simulink model "COSTEP_Auto"  (R2024b)
settings: Solver=FixedStepAuto  StartTime=0.0  StopTime=25  FixedStep=1/3600  RelTol=1e-3
model workspace (MAT data in the model file):
  AD : Simulink.Parameter (value not decoded)
  AG : Simulink.Parameter (value not decoded)
  AH : Simulink.Parameter (value not decoded)
  AV : Simulink.Parameter (value not decoded)
  AVP : Simulink.Parameter (value not decoded)
  BCHL : Simulink.Parameter (value not decoded)
  BCHV : Simulink.Parameter (value not decoded)
  BD : Simulink.Parameter (value not decoded)
  BG : Simulink.Parameter (value not decoded)
  BH : Simulink.Parameter (value not decoded)
  BVP : Simulink.Parameter (value not decoded)
  CD : Simulink.Parameter (value not decoded)
  CG : Simulink.Parameter (value not decoded)
  CH : Simulink.Parameter (value not decoded)
  CVP : Simulink.Parameter (value not decoded)
  ISV : Simulink.Parameter (value not decoded)
  XMW : Simulink.Parameter (value not decoded)
  XNS : Simulink.Parameter (value not decoded)
  XNS2 : Simulink.Parameter (value not decoded)
  XNS3 : Simulink.Parameter (value not decoded)
  XNSE : Simulink.Parameter (value not decoded)
values from neighbouring files (symbols this model uses):
  DD = SimData{4,1}{1,2}    [Auto_run_COSTEP.m]    (also in Run_COSTEP.m)
  G = SimData{2,1}(j,2)    [Auto_run_COSTEP.m]    (also in G.mat = [4243534565 7854912354 3456432354 1731738903 4346024432 5784; Run_COSTEP.m)
  IDV = SimData{3,1}(1:20,j)    [Auto_run_COSTEP.m]    (also in IDV.mat = [0 0 0 0 0 0 0 0 0 0 0 0 ... (812 elements, 28x29)]; Run_COSTEP.m = SimData{3,1}(1:28,j))
symbols that are objects in the model workspace (value not decoded): AD, AG, AH, AV, AVP, BD, BG, BH, BVP, CD, CG, CH, CVP, XMW, XNS, XNS2, XNS3, XNSE
undefined symbols (not defined in the file or in its folder): magnitude, msgbox, SETPT, XMEAS, XMV
libraries: mylib x304, dspindex x31
(part 7 of 13)

== system COSTEP_Auto/Stream Measurements/Subsystem6/E feed stream ==
  Stream 2 : Inport
  Bus Creator : BusCreator  Inputs=4
  Bus Selector : BusSelector  OutputSignals=XMNSE(3),XMNSE(4)
  Bus Selector1 : BusSelector  OutputSignals=TST(2),XST(I;2)
  Bus Selector2 : BusSelector  OutputSignals=Stream 2
  Bus Selector3 : BusSelector  OutputSignals=signal1.XMEAS(3)
  Composition measurement mol% : Subsystem
  Constant : Constant  Value=1000
  Flow measurement in kg/h : Subsystem
  Pressure measurement in kPa : Subsystem
  Temperature measurement in C : Subsystem
  tag scope: SM3=global
  wires:
  Bus Selector1/1 -> Temperature measurement in C/1(T in celsius)  "<TST(2)>"
  Temperature measurement in C/1(SMEAST(3)) -> Bus Creator/1  "SMEAST(3)"
  [XMNSE] -> Bus Selector/1
  Bus Selector/1 -> Temperature measurement in C/2(XMNSE)  "<XMNSE(3)>"
  Bus Selector/2 -> Pressure measurement in kPa/2(XMNSE)  "<XMNSE(4)>"
  Stream 2/1 -> Bus Selector1/1
  Bus Selector1/2 -> Composition measurement mol%/1(XST)  "<XST(I;2)>"
  Constant/1 -> Pressure measurement in kPa/1("P in mm Hg ")
  Pressure measurement in kPa/1(SMEASP(3)) -> Bus Creator/2  "SMEASP(3)"
  Flow measurement in kg/h/1("SMEASF(3) ") -> Bus Creator/3  "SMEASF(3)"
  Composition measurement mol%/1(SMEASX(3)) -> Bus Creator/4  "SMEASX(3)"
  Bus Creator/1 -> [SM3]
  [XMNSE2] -> Bus Selector2/1
  Bus Selector2/1 -> Composition measurement mol%/2(XMNSE)  "<Stream 2>"
  [XMEAS] -> Bus Selector3/1
  Bus Selector3/1 -> Flow measurement in kg/h/1(XMEAS in kg/h)  "<XMEAS(3)>"

== system COSTEP_Auto/Stream Measurements/Subsystem6/Product stream ==
  Stream 13 : Inport
  Bus Creator : BusCreator  Inputs=4
  Bus Selector : BusSelector  OutputSignals=XMNSE(14)
  Bus Selector1 : BusSelector  OutputSignals=PTC,XST(I;13)
  Bus Selector2 : BusSelector  OutputSignals=Stream 13
  Bus Selector3 : BusSelector  OutputSignals=signal4.XMEAS(18),signal4.XMEAS(17)
  Bus Selector4 : BusSelector  OutputSignals=Stream 13
  Composition measurement mol% : Subsystem
  Flow measurement in kg/h : Subsystem
  Pressure measurement in kPa : Subsystem
  Temperature measurement in C : Subsystem
  tag scope: SM11=global
  wires:
  Temperature measurement in C/1(SMEAST) -> Bus Creator/1
  [XMNSE] -> Bus Selector/1
  Stream 13/1 -> Bus Selector1/1
  Pressure measurement in kPa/1(SMEASP) -> Bus Creator/2
  Flow measurement in kg/h/1("SMEASF ") -> Bus Creator/3  "SMEASF"
  Composition measurement mol%/1(SMEASX) -> Bus Creator/4
  Bus Creator/1 -> [SM11]
  [XMNSE2] -> Bus Selector2/1
  Bus Selector2/1 -> Composition measurement mol%/2(XMNSE2)  "<Stream 13>"
  [XMEAS] -> Bus Selector3/1
  Bus Selector/1 -> Pressure measurement in kPa/2(XMNSE)  "<XMNSE(14)>"
  Bus Selector1/1 -> Pressure measurement in kPa/1("P in mm Hg ")  "<PTC>"
  Bus Selector3/1 -> Temperature measurement in C/1(XMEAS in celsius)  "<XMEAS(18)>"
  Bus Selector3/2 -> Flow measurement in kg/h/1(XMEAS in m^3/h)  "<XMEAS(17)>"
  Bus Selector1/2 -> Composition measurement mol%/1(XST), Flow measurement in kg/h/2(XST)  "<XST(I;13)>"
  [XMNSE3] -> Bus Selector4/1
  Bus Selector4/1 -> Composition measurement mol%/3(XMNSE3)  "<Stream 13>"

== system COSTEP_Auto/Stream Measurements/Subsystem6/Purge stream ==
  Stream 10 : Inport
  Bus Creator : BusCreator  Inputs=4
  Bus Selector : BusSelector  OutputSignals=XMNSE(2)
  Bus Selector1 : BusSelector  OutputSignals=signal1.XST(I;10)
  Bus Selector3 : BusSelector  OutputSignals=signal3.XMEAS(11),signal3.XMEAS(10),signal9
  Composition measurement mol% : Subsystem
  Flow measurement in kg/h : Subsystem
  Pressure measurement in kPa : Subsystem
  Temperature measurement in C : Subsystem
  tag scope: SM9=global
  wires:
  Temperature measurement in C/1(SMEAST) -> Bus Creator/1  "SMEAST"
  Stream 10/1 -> Bus Selector1/1
  Bus Selector1/1 -> Flow measurement in kg/h/2(XST)  "<XST(I;10)>"
  Pressure measurement in kPa/1(SMEASP) -> Bus Creator/2
  Flow measurement in kg/h/1("SMEASF ") -> Bus Creator/3  "SMEASF"
  Composition measurement mol%/1(SMEASX) -> Bus Creator/4
  Bus Creator/1 -> [SM9]
  [XMEAS] -> Bus Selector3/1
  Bus Selector3/1 -> Temperature measurement in C/1(XMEAS in celsius)  "<XMEAS(11)>"
  Bus Selector3/2 -> Flow measurement in kg/h/1(XMEAS in kscmh)  "<XMEAS(10)>"
  Bus Selector3/3 -> Composition measurement mol%/1(XMEAS)  "<signal9>"
  [XMNSE] -> Bus Selector/1
  Bus Selector/1 -> Pressure measurement in kPa/1(XMNSE)  "<XMNSE(2)>"

== system COSTEP_Auto/Stream Measurements/Subsystem6/RCIn ==
  Bus Creator : BusCreator  Inputs=3
  Bus Selector : BusSelector  OutputSignals=XMNSE(15),XMNSE(16),XMNSE(17)
  Flow measurement in kg/h : Subsystem
  Pressure measurement in kPa : Subsystem
  Temperature measurement in C : Subsystem
  tag scope: SM16=global
  wires:
  [TCWR] -> Pressure measurement in kPa/2(TC), Temperature measurement in C/1(T in celsius)
  [FWR] -> Flow measurement in kg/h/2(F in gpm)
  [XMNSE] -> Bus Selector/1
  Bus Selector/1 -> Temperature measurement in C/2(XMNSE)  "<XMNSE(15)>"
  Bus Selector/2 -> Pressure measurement in kPa/1(XMNSE)  "<XMNSE(16)>"
  Bus Selector/3 -> Flow measurement in kg/h/1(XMNSE)  "<XMNSE(17)>"
  Temperature measurement in C/1(SMEAST) -> Bus Creator/1
  Pressure measurement in kPa/1(SMEASP) -> Bus Creator/2
  Flow measurement in kg/h/1("SMEASF ") -> Bus Creator/3
  Bus Creator/1 -> [SM16]

== system COSTEP_Auto/Stream Measurements/Subsystem6/RCOut ==
  Bus Creator : BusCreator  Inputs=2
  Bus Selector : BusSelector  OutputSignals=XMNSE(18),XMNSE(19)
  Pressure measurement in kPa : Subsystem
  Temperature measurement in C : Subsystem
  tag scope: SM12=global
  wires:
  [TWR] -> Pressure measurement in kPa/2(TC), Temperature measurement in C/1(T in celsius)
  Bus Creator/1 -> [SM12]
  [XMNSE] -> Bus Selector/1
  Bus Selector/1 -> Temperature measurement in C/2(XMNSE)  "<XMNSE(18)>"
  Bus Selector/2 -> Pressure measurement in kPa/1(XMNSE)  "<XMNSE(19)>"
  Temperature measurement in C/1(SMEAST) -> Bus Creator/1
  Pressure measurement in kPa/1(SMEASP) -> Bus Creator/2

== system COSTEP_Auto/Stream Measurements/Subsystem6/Reactor feed stream ==
  Stream 6 : Inport
  Bus Creator : BusCreator  Inputs=4
  Bus Selector : BusSelector  OutputSignals=XMNSE(11)
  Bus Selector1 : BusSelector  OutputSignals=signal1.TST(6) = TST(7),signal1.XST(I;6) = XST(I;7)
  Bus Selector2 : BusSelector  OutputSignals=Stream 6
  Bus Selector3 : BusSelector  OutputSignals=signal4.XMEAS(16),signal2.XMEAS(6),signal8
  Composition measurement mol% : Subsystem
  Flow measurement in kg/h : Subsystem
  Pressure measurement in kPa : Subsystem
  Temperature measurement in C : Subsystem
  tag scope: SM6=global
  wires:
  Bus Selector1/1 -> Temperature measurement in C/1(T in celsius)  "<TST(6) = TST(7)>"
  Temperature measurement in C/1(SMEAST) -> Bus Creator/1  "SMEAST(6)"
  [XMNSE] -> Bus Selector/1
  Bus Selector/1 -> Temperature measurement in C/2(XMNSE)  "<XMNSE(11)>"
  Stream 6/1 -> Bus Selector1/1
  Bus Selector1/2 -> Flow measurement in kg/h/2(XST), Composition measurement mol%/1(XST)  "<XST(I;6) = XST(I;7)>"
  [XMEAS] -> Bus Selector3/1
  Pressure measurement in kPa/1(SMEASP) -> Bus Creator/2  "SMEASP(6)"
  Flow measurement in kg/h/1("SMEASF ") -> Bus Creator/3  "SMEASF(6)"
  Composition measurement mol%/1(SMEASX(6)) -> Bus Creator/4  "SMEASX(6)"
  Bus Creator/1 -> [SM6]
  [XMNSE2] -> Bus Selector2/1
  Bus Selector2/1 -> Composition measurement mol%/2(XMNSE)  "<Stream 6>"
  Bus Selector3/1 -> Pressure measurement in kPa/1(XMEAS in kPa gauge)  "<XMEAS(16)>"
  Bus Selector3/2 -> Flow measurement in kg/h/1(XMEAS in kscmh)  "<XMEAS(6)>"
  Bus Selector3/3 -> Composition measurement mol%/3(XMEAS)  "<signal8>"

== system COSTEP_Auto/Stream Measurements/Subsystem6/Reactor product stream ==
  Stream 8 : Inport
  Bus Creator : BusCreator  Inputs=4
  Bus Selector : BusSelector  OutputSignals=XMNSE(12)
  Bus Selector1 : BusSelector  OutputSignals=signal1.XST(I;8),signal1.FTM(8)
  Bus Selector2 : BusSelector  OutputSignals=Stream 8
  Bus Selector3 : BusSelector  OutputSignals=signal2.XMEAS(9),signal2.XMEAS(7)
  Composition measurement mol% : Subsystem
  Flow measurement in kg/h : Subsystem
  Pressure measurement in kPa : Subsystem
  Temperature measurement in C : Subsystem
  tag scope: SM7=global
  wires:
  Temperature measurement in C/1(SMEAST) -> Bus Creator/1
  [XMNSE] -> Bus Selector/1
  Stream 8/1 -> Bus Selector1/1
  Bus Selector1/1 -> Composition measurement mol%/1(XST), Flow measurement in kg/h/1(XST)  "<XST(I;8)>"
  Pressure measurement in kPa/1(SMEASP) -> Bus Creator/2
  Flow measurement in kg/h/1("SMEASF ") -> Bus Creator/3
  Composition measurement mol%/1(SMEASX) -> Bus Creator/4
  Bus Creator/1 -> [SM7]
  [XMNSE2] -> Bus Selector2/1
  Bus Selector2/1 -> Composition measurement mol%/2(XMNSE)  "<Stream 8>"
  [XMEAS] -> Bus Selector3/1
  Bus Selector3/1 -> Temperature measurement in C/1(XMEAS in celsius)  "<XMEAS(9)>"
  Bus Selector3/2 -> Pressure measurement in kPa/1(XMEAS in kPa gauge)  "<XMEAS(7)>"
  Bus Selector1/2 -> Flow measurement in kg/h/3(F in lb-mol/h)  "<FTM(8)>"
  Bus Selector/1 -> Flow measurement in kg/h/2(XMNSE)  "<XMNSE(12)>"

== system COSTEP_Auto/Stream Measurements/Subsystem6/Separator product stream ==
  Stream 9 : Inport
  Bus Creator : BusCreator  Inputs=4
  Bus Selector1 : BusSelector  OutputSignals=signal2.XST(I;9)
  Bus Selector2 : BusSelector  OutputSignals=Stream 9
  Bus Selector3 : BusSelector  OutputSignals=signal3.XMEAS(11),signal3.XMEAS(13),signal1.XMEAS(5),signal3.XMEAS(10)
  Composition measurement mol% : Subsystem
  Flow measurement in kg/h : Subsystem
  Pressure measurement in kPa : Subsystem
  Temperature measurement in C : Subsystem
  tag scope: SMNA=global
  wires:
  Temperature measurement in C/1(SMEAST) -> Bus Creator/1  "SMEAST"
  Stream 9/1 -> Bus Selector1/1
  Bus Selector1/1 -> Flow measurement in kg/h/2(XST), Composition measurement mol%/1(XST)  "<XST(I;9)>"
  Pressure measurement in kPa/1(SMEASP) -> Bus Creator/2
  Flow measurement in kg/h/1("SMEASF ") -> Bus Creator/3  "SMEASF"
  Composition measurement mol%/1(SMEASX) -> Bus Creator/4
  Bus Creator/1 -> [SMNA]
  [XMNSE2] -> Bus Selector2/1
  Bus Selector2/1 -> Composition measurement mol%/2(XMNSE)  "<Stream 9>"
  [XMEAS] -> Bus Selector3/1
  Bus Selector3/1 -> Temperature measurement in C/1(XMEAS in celsius)  "<XMEAS(11)>"
  Bus Selector3/2 -> Pressure measurement in kPa/1(XMEAS in kPa gauge)  "<XMEAS(13)>"
  Bus Selector3/3 -> Flow measurement in kg/h/1(XMEAS in kscmh)  "<XMEAS(5)>"
  Bus Selector3/4 -> Flow measurement in kg/h/3(XMEAS in kscmh1)  "<XMEAS(10)>"

== system COSTEP_Auto/Stream Measurements/Subsystem6/Separator recycle stream (after compressor) ==
  Stream 9 : Inport
  Bus Creator : BusCreator  Inputs=4
  Bus Selector1 : BusSelector  OutputSignals=signal2.XST(I;9),signal2.HST(9),signal2.Phase
  Bus Selector2 : BusSelector  OutputSignals=Stream 9
  Bus Selector3 : BusSelector  OutputSignals=signal4.XMEAS(16),signal1.XMEAS(5)
  Composition measurement mol% : Subsystem
  Flow measurement in kg/h : Subsystem
  Pressure measurement in kPa : Subsystem
  Temperature measurement in C : Subsystem
  tag scope: SM8=global
  wires:
  Temperature measurement in C/1(SMEAST) -> Bus Creator/1  "SMEAST"
  Stream 9/1 -> Bus Selector1/1
  Bus Selector1/1 -> Temperature measurement in C/2(XST), Flow measurement in kg/h/2(XST), Composition measurement mol%/1(XST)  "<XST(I;9)>"
  Pressure measurement in kPa/1(SMEASP) -> Bus Creator/2
  Flow measurement in kg/h/1("SMEASF ") -> Bus Creator/3  "SMEASF"
  Composition measurement mol%/1(SMEASX) -> Bus Creator/4
  Bus Creator/1 -> [SM8]
  [XMNSE2] -> Bus Selector2/1
  Bus Selector2/1 -> Composition measurement mol%/2(XMNSE)  "<Stream 9>"
  [XMEAS] -> Bus Selector3/1
  Bus Selector3/1 -> Pressure measurement in kPa/1(XMEAS in kPa gauge)  "<XMEAS(16)>"
  Bus Selector3/2 -> Flow measurement in kg/h/1(XMEAS in kscmh)  "<XMEAS(5)>"
  Bus Selector1/2 -> Temperature measurement in C/1(HST(9))  "<HST(9)>"
  Bus Selector1/3 -> Temperature measurement in C/3(ITY)  "<Phase>"

== system COSTEP_Auto/Stream Measurements/Subsystem6/Separator recycle stream (before compressor) ==
  Stream 9 : Inport
  Bus Creator : BusCreator  Inputs=4
  Bus Selector1 : BusSelector  OutputSignals=signal2.XST(I;9)
  Bus Selector2 : BusSelector  OutputSignals=Stream 9
  Bus Selector3 : BusSelector  OutputSignals=signal3.XMEAS(11),signal3.XMEAS(13),signal1.XMEAS(5)
  Composition measurement mol% : Subsystem
  Flow measurement in kg/h : Subsystem
  Pressure measurement in kPa : Subsystem
  Temperature measurement in C : Subsystem
  tag scope: SM15=global
  wires:
  Temperature measurement in C/1(SMEAST) -> Bus Creator/1  "SMEAST"
  Stream 9/1 -> Bus Selector1/1
  Bus Selector1/1 -> Flow measurement in kg/h/2(XST), Composition measurement mol%/1(XST)  "<XST(I;9)>"
  Pressure measurement in kPa/1(SMEASP) -> Bus Creator/2
  Flow measurement in kg/h/1("SMEASF ") -> Bus Creator/3  "SMEASF"
  Composition measurement mol%/1(SMEASX) -> Bus Creator/4
  Bus Creator/1 -> [SM15]
  [XMNSE2] -> Bus Selector2/1
  Bus Selector2/1 -> Composition measurement mol%/2(XMNSE)  "<Stream 9>"
  [XMEAS] -> Bus Selector3/1
  Bus Selector3/1 -> Temperature measurement in C/1(XMEAS in celsius)  "<XMEAS(11)>"
  Bus Selector3/2 -> Pressure measurement in kPa/1(XMEAS in kPa gauge)  "<XMEAS(13)>"
  Bus Selector3/3 -> Flow measurement in kg/h/1(XMEAS in kscmh)  "<XMEAS(5)>"

== system COSTEP_Auto/Stream Measurements/Subsystem6/Separator underflow stream ==
  Stream 11 : Inport
  Bus Creator : BusCreator  Inputs=4
  Bus Selector1 : BusSelector  OutputSignals=signal1.PTSL,signal1.XST(I;11)
  Bus Selector2 : BusSelector  OutputSignals=Stream 11
  Bus Selector3 : BusSelector  OutputSignals=signal3.XMEAS(11),signal3.XMEAS(14)
  Bus Selector4 : BusSelector  OutputSignals=XMNSE(13)
  Composition measurement mol% : Subsystem
  Flow measurement in kg/h : Subsystem
  Pressure measurement in kPa : Subsystem
  Temperature measurement in C : Subsystem
  tag scope: SM10=global
  wires:
  Temperature measurement in C/1(SMEAST) -> Bus Creator/1
  [XMNSE] -> Bus Selector4/1
  Stream 11/1 -> Bus Selector1/1
  Pressure measurement in kPa/1(SMEASP) -> Bus Creator/2
  Flow measurement in kg/h/1("SMEASF ") -> Bus Creator/3  "SMEASF"
  Composition measurement mol%/1(SMEASX) -> Bus Creator/4
  Bus Creator/1 -> [SM10]
  [XMNSE3] -> Bus Selector2/1
  Bus Selector2/1 -> Composition measurement mol%/2(XMNSE)  "<Stream 11>"
  [XMEAS] -> Bus Selector3/1
  Bus Selector4/1 -> Pressure measurement in kPa/2(XMNSE)  "<XMNSE(13)>"
  Bus Selector1/1 -> Pressure measurement in kPa/1("P in mm Hg ")  "<PTSL>"
  Bus Selector1/2 -> Flow measurement in kg/h/2(XST), Composition measurement mol%/1(XST)  "<XST(I;11)>"
  Bus Selector3/1 -> Temperature measurement in C/1(XMEAS in celsius)  "<XMEAS(11)>"
  Bus Selector3/2 -> Flow measurement in kg/h/1(XMEAS in m^3/h)  "<XMEAS(14)>"

== system COSTEP_Auto/Stream Measurements/Subsystem6/Stripper recycle stream ==
  Stream 5 : Inport
  Bus Creator : BusCreator  Inputs=4
  Bus Selector : BusSelector  OutputSignals=XMNSE(9),XMNSE(10)
  Bus Selector1 : BusSelector  OutputSignals=TST(5),XST(I;5),FTM(5)
  Bus Selector2 : BusSelector  OutputSignals=Stream 5
  Bus Selector3 : BusSelector  OutputSignals=signal4.XMEAS(16)
  Composition measurement mol% : Subsystem
  Flow measurement in kg/h : Subsystem
  Pressure measurement in kPa : Subsystem
  Temperature measurement in C : Subsystem
  tag scope: SM5=global
  wires:
  Bus Selector1/1 -> Temperature measurement in C/1(T in celsius)  "<TST(5)>"
  Temperature measurement in C/1(SMEAST(5)) -> Bus Creator/1  "SMEAST(5)"
  [XMNSE] -> Bus Selector/1
  Bus Selector/1 -> Temperature measurement in C/2(XMNSE)  "<XMNSE(9)>"
  Stream 5/1 -> Bus Selector1/1
  Bus Selector1/2 -> Composition measurement mol%/1(XST), Flow measurement in kg/h/1(XST)  "<XST(I;5)>"
  [XMEAS] -> Bus Selector3/1
  Pressure measurement in kPa/1(SMEASP(5)) -> Bus Creator/2  "SMEASP(5)"
  Flow measurement in kg/h/1("SMEASF(5) ") -> Bus Creator/3  "SMEASF(5)"
  Composition measurement mol%/1(SMEASX(5)) -> Bus Creator/4  "SMEASX(5)"
  Bus Creator/1 -> [SM5]
  [XMNSE2] -> Bus Selector2/1
  Bus Selector2/1 -> Composition measurement mol%/2(XMNSE)  "<Stream 5>"
  Bus Selector3/1 -> Pressure measurement in kPa/1(XMEAS in kPa gauge)  "<XMEAS(16)>"
  Bus Selector1/3 -> Flow measurement in kg/h/3(F in lb-mol/h)  "<FTM(5)>"
  Bus Selector/2 -> Flow measurement in kg/h/2(XMNSE)  "<XMNSE(10)>"

== system COSTEP_Auto/Stripper/Heat transfer of stripper/If Action Subsystem ==
  In1 : Inport
  Action Port : ActionPort  ActionPortLabel=if(u1 < 100)
  Out1 : Outport  VectorParamsAs1DForOutWhenUnconnected=off
  wires:
  In1/1 -> Out1/1

== system COSTEP_Auto/Stripper/Heat transfer of stripper/If Action Subsystem1 ==
  In1 : Inport
  Action Port : ActionPort  ActionPortLabel=else
  Out1 : Outport  VectorParamsAs1DForOutWhenUnconnected=off
  wires:
  In1/1 -> Out1/1

== system COSTEP_Auto/Stripper/Holdup of Components in Stripper/Holsup of Liquid Components in Stripper ==
  YY(19:26) : Inport
  Bus Creator : BusCreator  Inputs=8
  Bus Selector : BusSelector  OutputSignals=YY(19),YY(20),YY(21),YY(22),YY(23),YY(24),YY(25),YY(26)
  UCLC(1) Holdup of Component A (Liquid) in Stripper lb-mol : Gain
  UCLC(2) Holdup of Component B (Liquid) in Stripper lb-mol : Gain
  UCLC(3) Holdup of Component C (Liquid) in Stripper lb-mol : Gain
  UCLC(4) Holdup of Component D (Liquid) in Stripper lb-mol : Gain
  UCLC(5) Holdup of Component E (Liquid) in Stripper lb-mol : Gain
  UCLC(6) Holdup of Component F (Liquid) in Stripper lb-mol : Gain
  UCLC(7) Holdup of Component G (Liquid) in Stripper lb-mol : Gain
  UCLC(8) Holdup of Component H (Liquid) in Stripper lb-mol : Gain
  UCLC : Outport  VectorParamsAs1DForOutWhenUnconnected=off
  wires:
  UCLC(8) Holdup of Component H (Liquid) in Stripper lb-mol/1 -> Bus Creator/8
  UCLC(2) Holdup of Component B (Liquid) in Stripper lb-mol/1 -> Bus Creator/2
  UCLC(1) Holdup of Component A (Liquid) in Stripper lb-mol/1 -> Bus Creator/1
  Bus Creator/1 -> UCLC/1
  UCLC(5) Holdup of Component E (Liquid) in Stripper lb-mol/1 -> Bus Creator/5
  UCLC(7) Holdup of Component G (Liquid) in Stripper lb-mol/1 -> Bus Creator/7
  UCLC(4) Holdup of Component D (Liquid) in Stripper lb-mol/1 -> Bus Creator/4
  UCLC(6) Holdup of Component F (Liquid) in Stripper lb-mol/1 -> Bus Creator/6
  UCLC(3) Holdup of Component C (Liquid) in Stripper lb-mol/1 -> Bus Creator/3
  YY(19:26)/1 -> Bus Selector/1
  Bus Selector/1 -> UCLC(1) Holdup of Component A (Liquid) in Stripper lb-mol/1  "<YY(19)>"
  Bus Selector/2 -> UCLC(2) Holdup of Component B (Liquid) in Stripper lb-mol/1  "<YY(20)>"
  Bus Selector/3 -> UCLC(3) Holdup of Component C (Liquid) in Stripper lb-mol/1  "<YY(21)>"
  Bus Selector/4 -> UCLC(4) Holdup of Component D (Liquid) in Stripper lb-mol/1  "<YY(22)>"
  Bus Selector/5 -> UCLC(5) Holdup of Component E (Liquid) in Stripper lb-mol/1  "<YY(23)>"
  Bus Selector/6 -> UCLC(6) Holdup of Component F (Liquid) in Stripper lb-mol/1  "<YY(24)>"
  Bus Selector/7 -> UCLC(7) Holdup of Component G (Liquid) in Stripper lb-mol/1  "<YY(25)>"
  Bus Selector/8 -> UCLC(8) Holdup of Component H (Liquid) in Stripper lb-mol/1  "<YY(26)>"

== system COSTEP_Auto/Stripper/Holdup of Components in Stripper/Liquid Component Fraction in Stripper ==
  UTLC : Inport
  UCLC : Inport  Port=2
  Bus Selector : BusSelector  OutputSignals=signal1,signal2,signal3,signal4,signal5,signal6,signal7,signal8
  Mux : Mux  Inputs=8
  XLC(1) : Product  Inputs=*/
  XLC(2) : Product  Inputs=*/
  XLC(3) : Product  Inputs=*/
  XLC(4) : Product  Inputs=*/
  XLC(5) : Product  Inputs=*/
  XLC(6) : Product  Inputs=*/
  XLC(7) : Product  Inputs=*/
  XLC(8) : Product  Inputs=*/
  XLC : Outport  VectorParamsAs1DForOutWhenUnconnected=off
  wires:
  XLC(3)/1 -> Mux/3  "XLC(3)"
  Bus Selector/2 -> XLC(2)/1  "<signal2>"
  Bus Selector/7 -> XLC(7)/1  "<signal7>"
  XLC(5)/1 -> Mux/5  "XLC(5)"
  XLC(7)/1 -> Mux/7  "XLC(7)"
  Bus Selector/3 -> XLC(3)/1  "<signal3>"
  UTLC/1 -> XLC(8)/2, XLC(7)/2, XLC(6)/2, XLC(5)/2, XLC(4)/2, XLC(3)/2, XLC(2)/2, XLC(1)/2
  Bus Selector/6 -> XLC(6)/1  "<signal6>"
  Bus Selector/5 -> XLC(5)/1  "<signal5>"
  XLC(2)/1 -> Mux/2  "XLC(2)"
  XLC(6)/1 -> Mux/6  "XLC(6)"
  Bus Selector/4 -> XLC(4)/1  "<signal4>"
  XLC(1)/1 -> Mux/1  "XLC(1)"
  XLC(8)/1 -> Mux/8  "XLC(8)"
  UCLC/1 -> Bus Selector/1
  XLC(4)/1 -> Mux/4  "XLC(4)"
  Mux/1 -> XLC/1
  Bus Selector/1 -> XLC(1)/1  "<signal1>"
  Bus Selector/8 -> XLC(8)/1  "<signal8>"

== system COSTEP_Auto/Stripper/Holdup of Components in Stripper/YP(19) ==
  FCM(1,12) : Inport
  FCM(1,13) : Inport  Port=2
  " " : Sum  Inputs=+-
  Integration : mylib/Integration  SystemSampleTime=-1  VariantActivationTime=update diagram  AllowFlexibleInterface=on  Latency=0  AutoFrameSizeCalculation=off
  "YY(19) " : Constant  Value=0.4306056376
  YY(19) : Outport  VectorParamsAs1DForOutWhenUnconnected=off
  wires:
  "YY(19) "/1 -> Integration/2
  FCM(1,13)/1 -> " "/2
  FCM(1,12)/1 -> " "/1
  " "/1 -> Integration/1
  Integration/1 -> YY(19)/1

== system COSTEP_Auto/Stripper/Holdup of Components in Stripper/YP(20) ==
  FCM(2,12) : Inport
  FCM(2,13) : Inport  Port=2
  " " : Sum  Inputs=+-
  Integration : mylib/Integration  SystemSampleTime=-1  VariantActivationTime=update diagram  AllowFlexibleInterface=on  Latency=0  AutoFrameSizeCalculation=off
  "YY(20) " : Constant  Value=7.9906200783E-3
  YY(20) : Outport  VectorParamsAs1DForOutWhenUnconnected=off
  wires:
  Integration/1 -> YY(20)/1
  FCM(2,12)/1 -> " "/1
  FCM(2,13)/1 -> " "/2
  "YY(20) "/1 -> Integration/2
  " "/1 -> Integration/1

== system COSTEP_Auto/Stripper/Holdup of Components in Stripper/YP(21) ==
  FCM(3,12) : Inport
  FCM(3,13) : Inport  Port=2
  " " : Sum  Inputs=+-
  Integration : mylib/Integration  SystemSampleTime=-1  VariantActivationTime=update diagram  AllowFlexibleInterface=on  Latency=0  AutoFrameSizeCalculation=off
  "YY(21) " : Constant  Value=0.9056036089
  YY(21) : Outport  VectorParamsAs1DForOutWhenUnconnected=off
  wires:
  Integration/1 -> YY(21)/1
  FCM(3,12)/1 -> " "/1
  FCM(3,13)/1 -> " "/2
  " "/1 -> Integration/1
  "YY(21) "/1 -> Integration/2

== system COSTEP_Auto/Stripper/Holdup of Components in Stripper/YP(22) ==
  FCM(4,12) : Inport
  FCM(4,13) : Inport  Port=2
  " " : Sum  Inputs=+-
  Integration : mylib/Integration  SystemSampleTime=-1  VariantActivationTime=update diagram  AllowFlexibleInterface=on  Latency=0  AutoFrameSizeCalculation=off
  "YY(22) " : Constant  Value=1.6054258216E-2
  "YY(22)  " : Outport  VectorParamsAs1DForOutWhenUnconnected=off
  wires:
  Integration/1 -> "YY(22)  "/1
  FCM(4,12)/1 -> " "/1
  FCM(4,13)/1 -> " "/2
  " "/1 -> Integration/1
  "YY(22) "/1 -> Integration/2

== system COSTEP_Auto/Stripper/Holdup of Components in Stripper/YP(23) ==
  FCM(5,12) : Inport
  FCM(5,13) : Inport  Port=2
  " " : Sum  Inputs=+-
  Integration : mylib/Integration  SystemSampleTime=-1  VariantActivationTime=update diagram  AllowFlexibleInterface=on  Latency=0  AutoFrameSizeCalculation=off
  "YY(23) " : Constant  Value=0.7509759687
  "YY(23)  " : Outport  VectorParamsAs1DForOutWhenUnconnected=off
  wires:
  Integration/1 -> "YY(23)  "/1
  FCM(5,12)/1 -> " "/1
  FCM(5,13)/1 -> " "/2
  " "/1 -> Integration/1
  "YY(23) "/1 -> Integration/2

== system COSTEP_Auto/Stripper/Holdup of Components in Stripper/YP(24) ==
  FCM(6,12) : Inport
  FCM(6,13) : Inport  Port=2
  " " : Sum  Inputs=+-
  Integration : mylib/Integration  SystemSampleTime=-1  VariantActivationTime=update diagram  AllowFlexibleInterface=on  Latency=0  AutoFrameSizeCalculation=off
  YY(24) : Constant  Value=8.8582855955E-2
  "YY(24)  " : Outport  VectorParamsAs1DForOutWhenUnconnected=off
  wires:
  Integration/1 -> "YY(24)  "/1
  FCM(6,12)/1 -> " "/1
  FCM(6,13)/1 -> " "/2
  " "/1 -> Integration/1
  YY(24)/1 -> Integration/2

== system COSTEP_Auto/Stripper/Holdup of Components in Stripper/YP(25) ==
  FCM(7,12) : Inport
  FCM(7,13) : Inport  Port=2
  " " : Sum  Inputs=+-
  Integration : mylib/Integration  SystemSampleTime=-1  VariantActivationTime=update diagram  AllowFlexibleInterface=on  Latency=0  AutoFrameSizeCalculation=off
  "YY(25) " : Constant  Value=48.27726193
  "YY(25)  " : Outport  VectorParamsAs1DForOutWhenUnconnected=off
  wires:
  Integration/1 -> "YY(25)  "/1
  FCM(7,12)/1 -> " "/1
  FCM(7,13)/1 -> " "/2
  " "/1 -> Integration/1
  "YY(25) "/1 -> Integration/2

== system COSTEP_Auto/Stripper/Holdup of Components in Stripper/YP(26) ==
  FCM(8,12) : Inport
  FCM(8,13) : Inport  Port=2
  " " : Sum  Inputs=+-
  Integration : mylib/Integration  SystemSampleTime=-1  VariantActivationTime=update diagram  AllowFlexibleInterface=on  Latency=0  AutoFrameSizeCalculation=off
  "YY(26) " : Constant  Value=39.38459028
  "YY(26)   " : Outport  VectorParamsAs1DForOutWhenUnconnected=off
  wires:
  Integration/1 -> "YY(26)   "/1
  FCM(8,12)/1 -> " "/1
  FCM(8,13)/1 -> " "/2
  " "/1 -> Integration/1
  "YY(26) "/1 -> Integration/2

== system COSTEP_Auto/Stripper/PTC Pressure of Liquid zone in stripper mmHg/VPR Vapour Pressure mmHg ==
  TCR : Inport
  AVP(I) Antoine Coefficient A ln(mmHg) : Constant  Value=AVP
  Add : Sum
  Add1 : Sum
  BVP(I) Antoine Coefficient B ln(mmHg)·°C : Constant  Value=BVP
  CVP(I) Antoine Coefficient C °C : Constant  Value=CVP
  Divide : Product  Inputs=*/
  Math Function : Math  SignedPower=on
  VPR : Outport  VectorParamsAs1DForOutWhenUnconnected=off
  wires:
  BVP(I) Antoine Coefficient B ln(mmHg)·°C/1 -> Divide/1
  CVP(I) Antoine Coefficient C °C/1 -> Add/1
  AVP(I) Antoine Coefficient A ln(mmHg)/1 -> Add1/1
  Add/1 -> Divide/2
  Divide/1 -> Add1/2
  Add1/1 -> Math Function/1
  Math Function/1 -> VPR/1
  TCR/1 -> Add/2

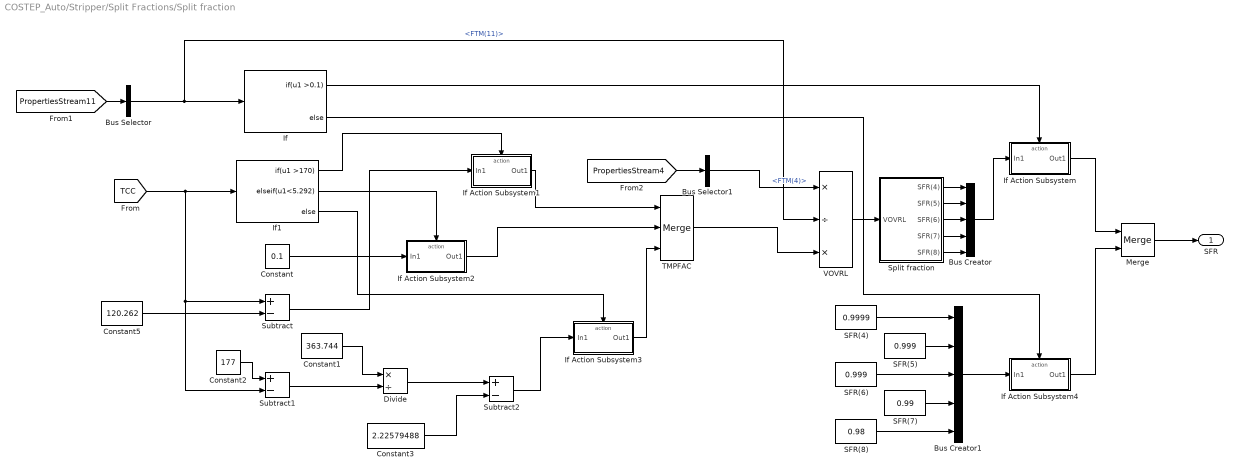
== system COSTEP_Auto/Stripper/Split Fractions/Split fraction ==
  Bus Creator : BusCreator  Inputs=5
  Bus Creator1 : BusCreator  Inputs=5
  Bus Selector : BusSelector  OutputSignals=signal1.FTM(11)
  Bus Selector1 : BusSelector  OutputSignals=FTM(4)
  Constant : Constant  Value=0.1
  Constant1 : Constant  Value=363.744
  Constant2 : Constant  Value=177
  Constant3 : Constant  Value=2.22579488
  Constant5 : Constant  Value=120.262
  Divide : Product  Inputs=*/
  If : If  IfExpression=u1 >0.1
  If Action Subsystem : Subsystem  TreatAsAtomicUnit=on
  If Action Subsystem1 : Subsystem  TreatAsAtomicUnit=on
  If Action Subsystem2 : Subsystem  TreatAsAtomicUnit=on
  If Action Subsystem3 : Subsystem  TreatAsAtomicUnit=on
  If Action Subsystem4 : Subsystem  TreatAsAtomicUnit=on
  If1 : If  IfExpression=u1 >170  ElseIfExpressions=u1<5.292
  Merge : Merge
  SFR(4) : Constant  Value=0.9999
  SFR(5) : Constant  Value=0.999
  SFR(6) : Constant  Value=0.999
  SFR(7) : Constant  Value=0.99
  SFR(8) : Constant  Value=0.98
  Split fraction : Subsystem
  Subtract : Sum  Inputs=+-
  Subtract1 : Sum  Inputs=+-
  Subtract2 : Sum  Inputs=+-
  "TMPFAC  " : Merge  Inputs=3
  VOVRL : Product  Inputs=*/*
  SFR : Outport  VectorParamsAs1DForOutWhenUnconnected=off
  wires:
  If/1 -> If Action Subsystem/Action
  Bus Selector/1 -> VOVRL/2, If/1  "<FTM(11)>"
  [TCC] -> If1/1, Subtract1/2, Subtract/1
  Constant5/1 -> Subtract/2
  Constant2/1 -> Subtract1/1
  Subtract1/1 -> Divide/2
  Constant1/1 -> Divide/1
  Divide/1 -> Subtract2/1
  Constant3/1 -> Subtract2/2
  If Action Subsystem1/1(Out1) -> "TMPFAC  "/1
  If Action Subsystem2/1(Out1) -> "TMPFAC  "/2
  If1/1 -> If Action Subsystem1/Action
  Subtract/1 -> If Action Subsystem1/1(In1)
  If1/2 -> If Action Subsystem2/Action
  Constant/1 -> If Action Subsystem2/1(In1)
  Subtract2/1 -> If Action Subsystem3/1(In1)
  If1/3 -> If Action Subsystem3/Action
  If Action Subsystem3/1(Out1) -> "TMPFAC  "/3
  Bus Selector1/1 -> VOVRL/1  "<FTM(4)>"
  "TMPFAC  "/1 -> VOVRL/3
  VOVRL/1 -> Split fraction/1(VOVRL)
  If/2 -> If Action Subsystem4/Action
  Split fraction/1(SFR(4)) -> Bus Creator/1
  Split fraction/2(SFR(5)) -> Bus Creator/2
  Split fraction/3(SFR(6)) -> Bus Creator/3
  Split fraction/4(SFR(7)) -> Bus Creator/4
  Split fraction/5(SFR(8)) -> Bus Creator/5
  Bus Creator/1 -> If Action Subsystem/1(In1)
  Bus Creator1/1 -> If Action Subsystem4/1(In1)
  SFR(4)/1 -> Bus Creator1/1
  SFR(5)/1 -> Bus Creator1/2
  SFR(6)/1 -> Bus Creator1/3
  SFR(7)/1 -> Bus Creator1/4
  SFR(8)/1 -> Bus Creator1/5
  If Action Subsystem4/1(Out1) -> Merge/2
  If Action Subsystem/1(Out1) -> Merge/1
  Merge/1 -> SFR/1
  [PropertiesStream11] -> Bus Selector/1
  [PropertiesStream4] -> Bus Selector1/1

== system COSTEP_Auto/Stripper/Stream 12/HST(12) Molar Enthalpy of Stream 12 MBtu//lb-mol ==
  ITY : Inport
  T : Inport  Port=2
  XST(I,I) : Inport  Port=3
  "Enthalpy of Stream " : mylib/Enthalpy of Stream   SystemSampleTime=-1  VariantActivationTime=update diagram  AllowFlexibleInterface=on  Latency=0  AutoFrameSizeCalculation=off
  "H " : Outport  VectorParamsAs1DForOutWhenUnconnected=off
  wires:
  ITY/1 -> "Enthalpy of Stream "/1
  T/1 -> "Enthalpy of Stream "/2
  XST(I,I)/1 -> "Enthalpy of Stream "/3
  "Enthalpy of Stream "/1 -> "H "/1

== system COSTEP_Auto/Stripper/Stream 13/HST(13) Molar Enthalpy of Stream 13 MBtu//lb-mol ==
  ITY : Inport
  T : Inport  Port=2
  XST(I,I) : Inport  Port=3
  "Enthalpy of Stream " : mylib/Enthalpy of Stream   SystemSampleTime=-1  VariantActivationTime=update diagram  AllowFlexibleInterface=on  Latency=0  AutoFrameSizeCalculation=off
  "H " : Outport  VectorParamsAs1DForOutWhenUnconnected=off
  wires:
  ITY/1 -> "Enthalpy of Stream "/1
  T/1 -> "Enthalpy of Stream "/2
  XST(I,I)/1 -> "Enthalpy of Stream "/3
  "Enthalpy of Stream "/1 -> "H "/1

== system COSTEP_Auto/Stripper/Stream 5/HST(5) Molar Enthalpy of Stream 5 MBtu//lb-mol ==
  ITY : Inport
  TST(5) : Inport  Port=2
  XST(I,5) : Inport  Port=3
  "Enthalpy of Stream " : mylib/Enthalpy of Stream   SystemSampleTime=-1  VariantActivationTime=update diagram  AllowFlexibleInterface=on  Latency=0  AutoFrameSizeCalculation=off
  "H " : Outport  PortDimensions=1  VectorParamsAs1DForOutWhenUnconnected=off
  wires:
  ITY/1 -> "Enthalpy of Stream "/1
  TST(5)/1 -> "Enthalpy of Stream "/2
  XST(I,5)/1 -> "Enthalpy of Stream "/3
  "Enthalpy of Stream "/1 -> "H "/1

== system COSTEP_Auto/Stripper/Volume of Stripper/DLC Molar Density of Liquids in Stripper lb-mol//ft³     ==
  XLC : Inport
  TCC : Inport  Port=2
  "DLC Molar Density of Liquids in Stripper lb-mol/ft³ " : Subsystem
  "DLC " : Outport  VectorParamsAs1DForOutWhenUnconnected=off
  wires:
  "DLC Molar Density of Liquids in Stripper lb-mol/ft³ "/1("R ") -> "DLC "/1
  TCC/1 -> "DLC Molar Density of Liquids in Stripper lb-mol/ft³ "/2(T)
  XLC/1 -> "DLC Molar Density of Liquids in Stripper lb-mol/ft³ "/1(X)

== system COSTEP_Auto/Valve/Position of Valve 1 %/Integration ==
  YP : Inport
  YY_0 : Inport  Port=2
  Integrator : Integrator  InitialConditionSource=external
  Subsystem : Subsystem
  YY : Outport
  wires:
  Subsystem/1(Out1) -> Integrator/1
  YP/1 -> Subsystem/1(In1)
  Integrator/1 -> YY/1
  YY_0/1 -> Integrator/2

== system COSTEP_Auto/Control Mode/Braatz/ /CONTROL 1 ==
  XMEAS(2) : Inport
  SETPT(1) : Inport  Port=2
  P Control Velocity form : mylib/Braatz Control/P Control Velocity form  Kc=GAIN1  Ts=SI1  X_0=XMV1_0  H=HIGH1
  XMV(1) : Outport  VectorParamsAs1DForOutWhenUnconnected=off
  wires:
  SETPT(1)/1 -> P Control Velocity form/1
  P Control Velocity form/1 -> XMV(1)/1
  XMEAS(2)/1 -> P Control Velocity form/2

== system COSTEP_Auto/Control Mode/Braatz/ /CONTROL 14 ==
  XMEAS(26) : Inport
  Constant : Constant  Value=SETPT14
  PI Control Setpoint Velocity form : Subsystem  mask{Kc=GAIN14, Ti=TAUI14, Ts=SI14, X_0=SETPT1, H=HIGH1, HS=HIGH14}
      mask prompts: Kc "Controller Gain - Kc"; Ti "Integral Time - Ti"; Ts "Sampling Interval - Ts"; X_0 "Initial Value"; H "High limit of measurment"; HS "High limit of setpoint"
      mask DialogControl DescGroupVar Prompt: Control Parameters
  SETPT(1) : Outport  VectorParamsAs1DForOutWhenUnconnected=off
  wires:
  Constant/1 -> PI Control Setpoint Velocity form/1(Setpoint)
  XMEAS(26)/1 -> PI Control Setpoint Velocity form/2(Measurement)
  PI Control Setpoint Velocity form/1(Output) -> SETPT(1)/1

== system COSTEP_Auto/Control Mode/Braatz/ 1/CONTROL 15 ==
  XMEAS(27) : Inport
  Constant : Constant  Value=SETPT15
  PI Control Setpoint Velocity form : mylib/Braatz Control/PI Control Setpoint Velocity form  Kc=GAIN15  Ti=TAUI15  Ts=SI15  X_0=SETPT2  H=HIGH2  HS=HIGH15
  SETPT(2) : Outport  VectorParamsAs1DForOutWhenUnconnected=off
  wires:
  Constant/1 -> PI Control Setpoint Velocity form/1
  XMEAS(27)/1 -> PI Control Setpoint Velocity form/2
  PI Control Setpoint Velocity form/1 -> SETPT(2)/1

== system COSTEP_Auto/Control Mode/Braatz/ 1/CONTROL 2 ==
  XMEAS(2) : Inport
  SETPT(2) : Inport  Port=2
  P Control Velocity form : mylib/Braatz Control/P Control Velocity form  Kc=GAIN2  Ts=SI2  X_0=XMV2_0  H=HIGH2
  XMV(2) : Outport  VectorParamsAs1DForOutWhenUnconnected=off
  wires:
  SETPT(2)/1 -> P Control Velocity form/1
  P Control Velocity form/1 -> XMV(2)/1
  XMEAS(2)/1 -> P Control Velocity form/2

== system COSTEP_Auto/Control Mode/Braatz/ 10/CONTROL 19 ==
  XMEAS(30) : Inport
  Constant : Constant  Value=SETPT19
  PI Control Setpoint Velocity form : mylib/Braatz Control/PI Control Setpoint Velocity form  Kc=GAIN19  Ti=TAUI19  Ts=SI19  X_0=SETPT6  H=HIGH6  HS=HIGH19
  SETPT(6) : Outport  VectorParamsAs1DForOutWhenUnconnected=off
  wires:
  Constant/1 -> PI Control Setpoint Velocity form/1
  XMEAS(30)/1 -> PI Control Setpoint Velocity form/2
  PI Control Setpoint Velocity form/1 -> SETPT(6)/1

== system COSTEP_Auto/Control Mode/Braatz/ 10/CONTROL 6 ==
  SETPT(6) : Inport
  XMEAS : Inport  Port=2
  Bus Selector : BusSelector  OutputSignals=signal3.XMEAS(10)
  P Control Velocity form : Subsystem  mask{Kc=GAIN6, Ts=SI6, X_0=XMV6_0, H=HIGH6}
      mask prompts: Kc "Controller Gain - Kc"; Ts "Sampling Interval - Ts"; X_0 "Initial Value"; H "High Limit of measurement"
      mask DialogControl DescGroupVar Prompt: Control Parameters
  XMV(6) : Outport  VectorParamsAs1DForOutWhenUnconnected=off
  wires:
  SETPT(6)/1 -> P Control Velocity form/1(Setpoint)
  P Control Velocity form/1(Output) -> XMV(6)/1
  Bus Selector/1 -> P Control Velocity form/2(Measurement)  "<XMEAS(10)>"
  XMEAS/1 -> P Control Velocity form/3(XMEAS), Bus Selector/1

== system COSTEP_Auto/Control Mode/Braatz/ 2/CONTROL 13 ==
  XMEAS(23) : Inport
  Constant : Constant  Value=SETPT13
  PI Control Setpoint Velocity form : mylib/Braatz Control/PI Control Setpoint Velocity form  Kc=GAIN13  Ti=TAUI13  Ts=SI13  X_0=SETPT3  H=HIGH3  HS=HIGH13
  SETPT(3) : Outport  VectorParamsAs1DForOutWhenUnconnected=off
  wires:
  Constant/1 -> PI Control Setpoint Velocity form/1
  XMEAS(23)/1 -> PI Control Setpoint Velocity form/2
  PI Control Setpoint Velocity form/1 -> SETPT(3)/1

== system COSTEP_Auto/Control Mode/Braatz/ 2/CONTROL 3 ==
  XMEAS(1) : Inport
  SETPT(3) : Inport  Port=2
  P Control Velocity form : mylib/Braatz Control/P Control Velocity form  Kc=GAIN3  Ts=SI3  X_0=XMV3_0  H=HIGH3
  XMV(3) : Outport
  wires:
  XMEAS(1)/1 -> P Control Velocity form/2
  P Control Velocity form/1 -> XMV(3)/1
  SETPT(3)/1 -> P Control Velocity form/1

== system COSTEP_Auto/Control Mode/Braatz/ 3/CONTROL 17 ==
  XMEAS(8) : Inport
  Constant : Constant  Value=SETPT17
  PI Control Setpoint Velocity form : Subsystem  AncestorBlock=|  mask{Kc=GAIN17, Ti=TAUI17, Ts=SI17, X_0=SETPT4, H=HIGH4, HS=HIGH17}
      | mylib/Braatz Control/PI Control
      | Setpoint
      | Velocity form
      mask prompts: Kc "Controller Gain - Kc"; Ti "Integral Time - Ti"; Ts "Sampling Interval - Ts"; X_0 "Initial Value"; H "High limit of measurment"; HS "High limit of setpoint"
      mask DialogControl DescGroupVar Prompt: Control Parameters
  SETPT(4) : Outport  VectorParamsAs1DForOutWhenUnconnected=off
  wires:
  Constant/1 -> PI Control Setpoint Velocity form/1(Setpoint)
  XMEAS(8)/1 -> PI Control Setpoint Velocity form/2(Measurement)
  PI Control Setpoint Velocity form/1(Output) -> SETPT(4)/1

== system COSTEP_Auto/Control Mode/Braatz/ 3/CONTROL 4 ==
  XMEAS(4) : Inport
  SETPT(4) : Inport  Port=2
  P Control Velocity form : mylib/Braatz Control/P Control Velocity form  Kc=GAIN4  Ts=SI4  X_0=XMV4_0  H=HIGH4
  XMV(4) : Outport  VectorParamsAs1DForOutWhenUnconnected=off
  wires:
  P Control Velocity form/1 -> XMV(4)/1
  XMEAS(4)/1 -> P Control Velocity form/2
  SETPT(4)/1 -> P Control Velocity form/1

== system COSTEP_Auto/Control Mode/Braatz/ 4/CONTROL 5 ==
  XMEAS(5) : Inport
  Constant4 : Constant  Value=SETPT5
  PI Control Measurement Velocity form : mylib/Braatz Control/PI Control Measurement Velocity form  Kc=GAIN5  Ti=TAUI5  Ts=SI5  X_0=XMV5_0  H=HIGH5
  XMV(5) : Outport  VectorParamsAs1DForOutWhenUnconnected=off
  wires:
  XMEAS(5)/1 -> PI Control Measurement Velocity form/2
  PI Control Measurement Velocity form/1 -> XMV(5)/1
  Constant4/1 -> PI Control Measurement Velocity form/1

== system COSTEP_Auto/Control Mode/Braatz/ 5/CONTROL 7 ==
  XMEAS(12) : Inport
  Constant4 : Constant  Value=SETPT7
  P Control Velocity form : mylib/Braatz Control/P Control Velocity form  Kc=GAIN7  Ts=SI7  X_0=XMV7_0  H=HIGH7
  XMV(7) : Outport  VectorParamsAs1DForOutWhenUnconnected=off
  wires:
  P Control Velocity form/1 -> XMV(7)/1
  Constant4/1 -> P Control Velocity form/1
  XMEAS(12)/1 -> P Control Velocity form/2

== system COSTEP_Auto/Control Mode/Braatz/ 6/CONTROL 8 ==
  XMEAS(15) : Inport
  Constant4 : Constant  Value=SETPT8
  P Control Velocity form : mylib/Braatz Control/P Control Velocity form  Kc=GAIN8  Ts=SI8  X_0=XMV8_0  H=HIGH8
  XMV(8) : Outport  VectorParamsAs1DForOutWhenUnconnected=off
  wires:
  P Control Velocity form/1 -> XMV(8)/1
  Constant4/1 -> P Control Velocity form/1
  XMEAS(15)/1 -> P Control Velocity form/2

== system COSTEP_Auto/Control Mode/Braatz/ 7/CONTROL 11 ==
  XMEAS(17) : Inport
  Constant4 : Constant  Value=SETPT11
  PI Control Measurement Velocity form : mylib/Braatz Control/PI Control Measurement Velocity form  Kc=GAIN11  Ti=TAUI11  Ts=SI11  X_0=XMV11_0  H=HIGH11
  XMV(11) : Outport  VectorParamsAs1DForOutWhenUnconnected=off
  wires:
  PI Control Measurement Velocity form/1 -> XMV(11)/1
  Constant4/1 -> PI Control Measurement Velocity form/1
  XMEAS(17)/1 -> PI Control Measurement Velocity form/2

== system COSTEP_Auto/Control Mode/Braatz/ 8/CONTROL 10 ==
  XMEAS(21) : Inport
  SETPT(10) : Inport  Port=2
  PI Control Measurement Velocity form : mylib/Braatz Control/PI Control Measurement Velocity form  Kc=GAIN10  Ti=TAUI10  Ts=SI10  X_0=XMV10_0  H=HIGH10
  XMV(10) : Outport  VectorParamsAs1DForOutWhenUnconnected=off
  wires:
  PI Control Measurement Velocity form/1 -> XMV(10)/1
  SETPT(10)/1 -> PI Control Measurement Velocity form/1
  XMEAS(21)/1 -> PI Control Measurement Velocity form/2

== system COSTEP_Auto/Control Mode/Braatz/ 8/CONTROL 18 ==
  XMEAS(9) : Inport
  Constant : Constant  Value=SETPT18
  PI Control Setpoint Velocity form : Subsystem  AncestorBlock=|  mask{Kc=GAIN18, Ti=TAUI18, Ts=SI18, X_0=SETPT10, H=HIGH10, HS=HIGH18}
      | mylib/Braatz Control/PI Control
      | Setpoint
      | Velocity form
      mask prompts: Kc "Controller Gain - Kc"; Ti "Integral Time - Ti"; Ts "Sampling Interval - Ts"; X_0 "Initial Value"; H "High limit of measurment"; HS "High limit of setpoint"
      mask DialogControl DescGroupVar Prompt: Control Parameters
  SETPT(10) : Outport  VectorParamsAs1DForOutWhenUnconnected=off
  wires:
  Constant/1 -> PI Control Setpoint Velocity form/1(Setpoint)
  XMEAS(9)/1 -> PI Control Setpoint Velocity form/2(Measurement)
  PI Control Setpoint Velocity form/1(Output) -> SETPT(10)/1

== system COSTEP_Auto/Control Mode/Braatz/ 9/CONTROL 16 ==
  XMEAS(18) : Inport
  SETPT(16) : Inport  Port=2
  PI Control Setpoint Velocity form : mylib/Braatz Control/PI Control Setpoint Velocity form  Kc=GAIN16  Ti=TAUI16  Ts=SI16  X_0=SETPT9  H=HIGH9  HS=HIGH16
  SETPT(9) : Outport  VectorParamsAs1DForOutWhenUnconnected=off
  wires:
  SETPT(16)/1 -> PI Control Setpoint Velocity form/1
  XMEAS(18)/1 -> PI Control Setpoint Velocity form/2
  PI Control Setpoint Velocity form/1 -> SETPT(9)/1

== system COSTEP_Auto/Control Mode/Braatz/ 9/CONTROL 20 ==
  XMEAS(38) : Inport
  Constant : Constant  Value=SETPT20
  PI Control Setpoint Velocity form : mylib/Braatz Control/PI Control Setpoint Velocity form  Kc=GAIN20  Ti=TAUI20  Ts=SI20  X_0=SETPT16  H=HIGH16  HS=HIGH20
  SETPT(16) : Outport  VectorParamsAs1DForOutWhenUnconnected=off
  wires:
  Constant/1 -> PI Control Setpoint Velocity form/1
  XMEAS(38)/1 -> PI Control Setpoint Velocity form/2
  PI Control Setpoint Velocity form/1 -> SETPT(16)/1

== system COSTEP_Auto/Control Mode/Braatz/ 9/CONTROL 9 ==
  XMEAS(19) : Inport
  SETPT(9) : Inport  Port=2
  P Control Velocity form : mylib/Braatz Control/P Control Velocity form  Kc=GAIN9  Ts=SI9  X_0=XMV9_0  H=HIGH9
  XMV(9) : Outport  VectorParamsAs1DForOutWhenUnconnected=off
  wires:
  SETPT(9)/1 -> P Control Velocity form/1
  P Control Velocity form/1 -> XMV(9)/1
  XMEAS(19)/1 -> P Control Velocity form/2

== system COSTEP_Auto/Control Mode/Ricker/Subsystem/Control Loop 1 ==
  Ratio 1 : Inport
  XMEAS(1) : Inport  Port=2
  Fp : Inport  Port=3
  PI Control Measurement Velocity form : mylib/Ricker/PI Control Measurement Velocity form  Kc=GAIN1  Ti=TAUI1  Ts=SI1  X_0=XMV3_0
  Product : Product
  XMV(3) : Outport
  wires:
  XMEAS(1)/1 -> PI Control Measurement Velocity form/2
  PI Control Measurement Velocity form/1 -> XMV(3)/1
  Product/1 -> PI Control Measurement Velocity form/1
  Ratio 1/1 -> Product/1
  Fp/1 -> Product/2

== system COSTEP_Auto/Control Mode/Ricker/Subsystem1/Control Loop 2 ==
  Ratio 2 : Inport
  XMEAS(2) : Inport  Port=2
  Fp : Inport  Port=3
  PI Control Measurement Velocity form : mylib/Ricker/PI Control Measurement Velocity form  Kc=GAIN2  Ti=TAUI2  Ts=SI2  X_0=XMV1_0
  Product : Product
  XMV(1) : Outport
  wires:
  XMEAS(2)/1 -> PI Control Measurement Velocity form/2
  PI Control Measurement Velocity form/1 -> XMV(1)/1
  Product/1 -> PI Control Measurement Velocity form/1
  Ratio 2/1 -> Product/1
  Fp/1 -> Product/2

== system COSTEP_Auto/Control Mode/Ricker/Subsystem2/Control Loop 3 ==
  Ratio 3 : Inport
  XMEAS(3) : Inport  Port=2
  Fp : Inport  Port=3
  PI Control Measurement Velocity form : mylib/Ricker/PI Control Measurement Velocity form  Kc=GAIN3  Ti=TAUI3  Ts=SI3  X_0=XMV3_0
  Product : Product
  XMV(2) : Outport
  wires:
  XMEAS(3)/1 -> PI Control Measurement Velocity form/2
  PI Control Measurement Velocity form/1 -> XMV(2)/1
  Product/1 -> PI Control Measurement Velocity form/1
  Ratio 3/1 -> Product/1
  Fp/1 -> Product/2

== system COSTEP_Auto/Control Mode/Ricker/Subsystem3/Control Loop 16 ==
  XMEAS(9) : Inport
  PI Control Measurement Velocity form : mylib/Ricker/PI Control Measurement Velocity form  Kc=GAIN16  Ti=TAUI16  Ts=SI16  X_0=XMV10_0
  Setpoint : Constant  Value=SETPT16
  XMV(10) : Outport
  wires:
  XMEAS(9)/1 -> PI Control Measurement Velocity form/2
  PI Control Measurement Velocity form/1 -> XMV(10)/1
  Setpoint/1 -> PI Control Measurement Velocity form/1

== system COSTEP_Auto/Control Mode/Ricker/Subsystem4/Control Loop 4 ==
  Ratio 4 : Inport
  XMEAS(4) : Inport  Port=2
  Fp : Inport  Port=3
  PI Control Measurement Velocity form : mylib/Ricker/PI Control Measurement Velocity form  Kc=GAIN4  Ti=TAUI4  Ts=SI4  X_0=XMV4_0
  Product : Product
  XMV(4) : Outport
  wires:
  XMEAS(4)/1 -> PI Control Measurement Velocity form/2
  PI Control Measurement Velocity form/1 -> XMV(4)/1
  Product/1 -> PI Control Measurement Velocity form/1
  Ratio 4/1 -> Product/1
  Fp/1 -> Product/2

== system COSTEP_Auto/Control Mode/Ricker/Subsystem5/Control Loop 12 ==
  XMEAS(7) : Inport
  Constant : Constant  Value=SETPT12
  PI Control Measurement Velocity form : mylib/Ricker/PI Control Measurement Velocity form  Kc=GAIN12  Ti=TAUI12  Ts=SI12  X_0=0.0034
  Ratio 5 : Outport
  wires:
  XMEAS(7)/1 -> PI Control Measurement Velocity form/2
  PI Control Measurement Velocity form/1 -> Ratio 5/1
  Constant/1 -> PI Control Measurement Velocity form/1

== system COSTEP_Auto/Control Mode/Ricker/Subsystem5/Control Loop 5 ==
  Ratio 5 : Inport
  XMEAS(10) : Inport  Port=2
  Fp : Inport  Port=3
  PI Control Measurement Velocity form : mylib/Ricker/PI Control Measurement Velocity form  Kc=GAIN5  Ti=TAUI5  Ts=SI5  X_0=XMV6_0
  Product : Product
  XMV(6) : Outport
  wires:
  XMEAS(10)/1 -> PI Control Measurement Velocity form/2
  PI Control Measurement Velocity form/1 -> XMV(6)/1
  Product/1 -> PI Control Measurement Velocity form/1
  Ratio 5/1 -> Product/1
  Fp/1 -> Product/2

== system COSTEP_Auto/Control Mode/Ricker/Subsystem6/Control Loop 10 ==
  XMEAS(12) : Inport
  Constant : Constant  Value=SETPT10
  PI Control Measurement Velocity form : mylib/Ricker/PI Control Measurement Velocity form  Kc=GAIN10  Ti=TAUI10  Ts=SI10  X_0=0.2516
  Ratio 6 : Outport
  wires:
  XMEAS(12)/1 -> PI Control Measurement Velocity form/2
  PI Control Measurement Velocity form/1 -> Ratio 6/1
  Constant/1 -> PI Control Measurement Velocity form/1

== system COSTEP_Auto/Control Mode/Ricker/Subsystem6/Control Loop 6 ==
  Ratio 6 : Inport
  XMEAS(14) : Inport  Port=2
  Fp : Inport  Port=3
  PI Control Measurement Velocity form : mylib/Ricker/PI Control Measurement Velocity form  Kc=GAIN6  Ti=TAUI6  Ts=SI6  X_0=XMV7_0
  Product : Product
  XMV(7) : Outport
  wires:
  XMEAS(14)/1 -> PI Control Measurement Velocity form/2
  PI Control Measurement Velocity form/1 -> XMV(7)/1
  Product/1 -> PI Control Measurement Velocity form/1
  Ratio 6/1 -> Product/1
  Fp/1 -> Product/2

== system COSTEP_Auto/Control Mode/Ricker/Subsystem7/Control Loop 7 ==
  Ratio 7 : Inport
  XMEAS(17) : Inport  Port=2
  Fp : Inport  Port=3
  PI Control Measurement Velocity form : mylib/Ricker/PI Control Measurement Velocity form  Kc=GAIN7  Ti=TAUI7  Ts=SI7  X_0=XMV8_0
  Product : Product
  XMV(8) : Outport
  wires:
  XMEAS(17)/1 -> PI Control Measurement Velocity form/2
  PI Control Measurement Velocity form/1 -> XMV(8)/1
  Product/1 -> PI Control Measurement Velocity form/1
  Ratio 7/1 -> Product/1
  Fp/1 -> Product/2

== system COSTEP_Auto/Control Mode/Ricker/Subsystem7/Control Loop 9 ==
  XMEAS(15) : Inport
  Constant : Constant  Value=SETPT9
  PI Control Measurement Velocity form : mylib/Ricker/PI Control Measurement Velocity form  Kc=GAIN9  Ti=TAUI9  Ts=SI9  X_0=0.2295
  Ratio 7 : Outport
  wires:
  XMEAS(15)/1 -> PI Control Measurement Velocity form/2
  PI Control Measurement Velocity form/1 -> Ratio 7/1
  Constant/1 -> PI Control Measurement Velocity form/1

== system COSTEP_Auto/Control Mode/Ricker/Subsystem8/Control Loop 11 ==
  XMEAS(8) : Inport
  PI Control Measurement Velocity form : Subsystem  AncestorBlock=|  mask{Kc=GAIN11, Ti=TAUI11, Ts=SI11, X_0=SETPT17}
      | mylib/Ricker/PI Control
      | Measurement
      | Velocity form
      mask prompts: Kc "Controller Gain - Kc"; Ti "Integral Time - Ti"; Ts "Sampling Interval - Ts"; X_0 "Initial Value"
      mask DialogControl DescGroupVar Prompt: Control Parameters
  Setpoint : Constant  Value=SETPT11
  SETPT17 : Outport
  wires:
  XMEAS(8)/1 -> PI Control Measurement Velocity form/2(Measurement)
  PI Control Measurement Velocity form/1(Output) -> SETPT17/1
  Setpoint/1 -> PI Control Measurement Velocity form/1(Setpoint)

== system COSTEP_Auto/Control Mode/Ricker/Subsystem8/Control Loop 17 ==
  XMEAS(11) : Inport
  SETPT17 : Inport  Port=2
  PI Control Measurement Velocity form : mylib/Ricker/PI Control Measurement Velocity form  Kc=GAIN17  Ti=TAUI17  Ts=SI17  X_0=XMV11_0
  XMV(11) : Outport
  wires:
  XMEAS(11)/1 -> PI Control Measurement Velocity form/2
  PI Control Measurement Velocity form/1 -> XMV(11)/1
  SETPT17/1 -> PI Control Measurement Velocity form/1

== system COSTEP_Auto/Mixing Zone/Stream 6/Subsystem/If Action Subsystem ==
  In1 : Inport
  Action Port : ActionPort  ActionPortLabel=if(u1 < 0)
  Out1 : Outport  VectorParamsAs1DForOutWhenUnconnected=off
  wires:
  In1/1 -> Out1/1
